simulink model "Limpert_Ex71"  (R2022a)
settings: Solver=FixedStepAuto  StartTime=0.0  StopTime=5  FixedStep=0.001  RelTol=1e-3
settings Model: Creator=roger  LastModifiedBy=wenis

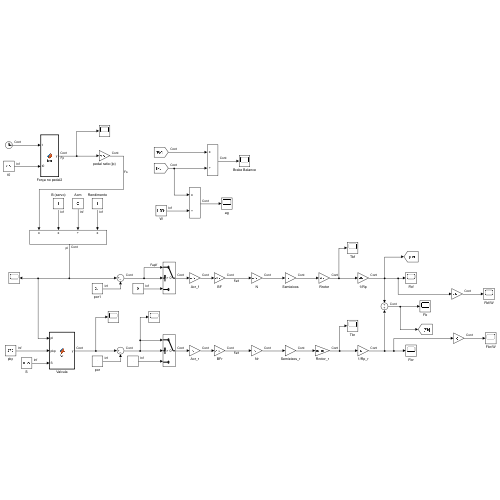
[thumbnail: Simulink's stored preview of the top-level diagram]
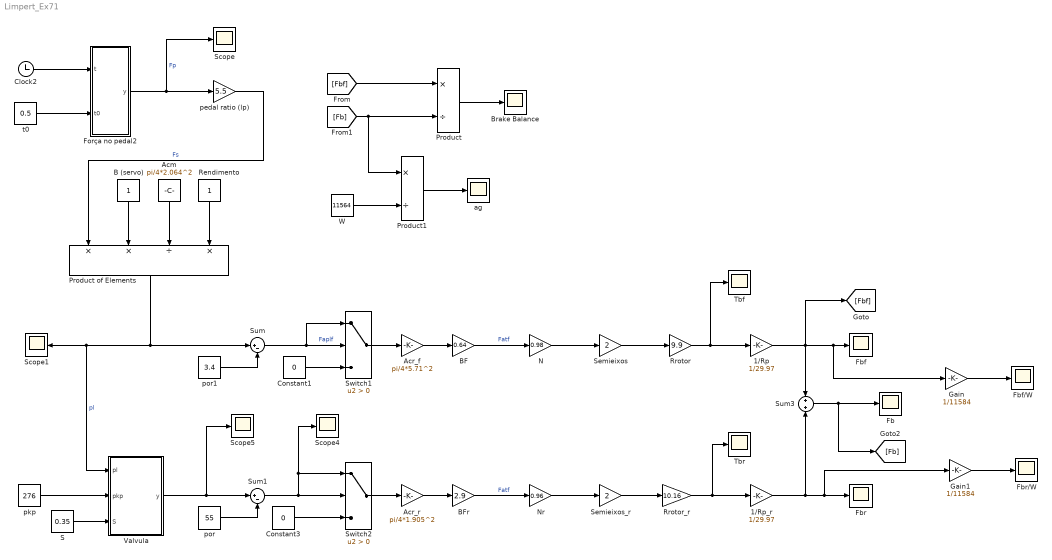
== system Limpert_Ex71 ==
  1/Rp : Gain  Gain=1/29.97
  1/Rp_r : Gain  Gain=1/29.97
  Acm : Constant  Value=pi/4*2.064^2
  Acr_f : Gain  Gain=pi/4*5.71^2
  Acr_r : Gain  Gain=pi/4*1.905^2
  B (servo) : Constant
  BF : Gain  Gain=0.64
  BFr : Gain  Gain=2.9
  Brake Balance : Scope
  Clock2 : Clock
  Constant1 : Constant  Value=0
  Constant3 : Constant  Value=0
  Fb : Scope
  Fbf : Scope
  Fbf/W : Scope
  Fbr : Scope
  Fbr/W : Scope
  Força no pedal2 : MATLAB Function  TreatAsAtomicUnit=on
  Gain : Gain  Gain=1/11584
  Gain1 : Gain  Gain=1/11584
  N : Gain  Gain=0.98
  Nr : Gain  Gain=0.96
  Product : Product  Inputs=*/
  Product of Elements : Product  Inputs=**/*
  Product1 : Product  Inputs=*/
  Rendimento : Constant
  Rrotor : Gain  Gain=9.9
  Rrotor_r : Gain  Gain=10.16
  S : Constant  Value=0.35
  Scope{,1,4..5} (4 alike) : Scope
  Semieixos : Gain  Gain=2
  Semieixos_r : Gain  Gain=2
  Sum : Sum  Inputs=|+-
  Sum1 : Sum  Inputs=|+-
  Sum3 : Sum
  Switch1 : Switch  Criteria=u2 > Threshold  SaturateOnIntegerOverflow=off  InputSameDT=off
  Switch2 : Switch  Criteria=u2 > Threshold  SaturateOnIntegerOverflow=off  InputSameDT=off
  Tbf : Scope
  Tbr : Scope
  Valvula : MATLAB Function  TreatAsAtomicUnit=on
  W : Constant  Value=11564
  ag : Scope
  pedal ratio (lp) : Gain  Gain=5.5
  pkp : Constant  Value=276
  por : Constant  Value=55
  por1 : Constant  Value=3.4
  t0 : Constant  Value=0.5
  wires:
  pedal ratio (lp)/1 -> Product of Elements/1  "Fs"
  B (servo)/1 -> Product of Elements/2
  Acm/1 -> Product of Elements/3
  Rendimento/1 -> Product of Elements/4
  pkp/1 -> Valvula/2(pkp)
  Sum/1 -> Switch1/1, Switch1/2  "Faplf"
  Acr_f/1 -> BF/1
  BF/1 -> N/1  "Fatf"
  N/1 -> Semieixos/1
  Semieixos/1 -> Rrotor/1
  Rrotor/1 -> Tbf/1, 1/Rp/1
  1/Rp/1 -> [Fbf], Sum3/1, Gain/1, Fbf/1
  1/Rp_r/1 -> Sum3/2, Gain1/1, Fbr/1
  Rrotor_r/1 -> 1/Rp_r/1, Tbr/1
  Semieixos_r/1 -> Rrotor_r/1
  Nr/1 -> Semieixos_r/1
  BFr/1 -> Nr/1  "Fatf"
  Acr_r/1 -> BFr/1
  Sum1/1 -> Switch2/2, Switch2/1, Scope4/1
  Sum3/1 -> [Fb], Fb/1
  S/1 -> Valvula/3(S)
  Valvula/1(y) -> Sum1/1, Scope5/1
  Constant3/1 -> Switch2/3
  por/1 -> Sum1/2
  Switch2/1 -> Acr_r/1
  por1/1 -> Sum/2
  Switch1/1 -> Acr_f/1
  Constant1/1 -> Switch1/3
  Product of Elements/1 -> Scope1/1, Valvula/1(pl), Sum/1  "pl"
  Clock2/1 -> Força no pedal2/1(t)
  t0/1 -> Força no pedal2/2(t0)
  Força no pedal2/1(y) -> Scope/1, pedal ratio (lp)/1  "Fp"
  [Fbf] -> Product/1
  [Fb] -> Product1/1, Product/2
  Product/1 -> Brake Balance/1
  W/1 -> Product1/2
  Product1/1 -> ag/1
  Gain/1 -> Fbf/W/1
  Gain1/1 -> Fbr/W/1

== matlab function Limpert_Ex71/Valvula ==
  data: pl input; y output; pkp input; S input
function y = fcn(pl, pkp, S)



if pl <= pkp
    y = pl;
else
    y = pkp + S*(pl-pkp);
end

end

== matlab function Limpert_Ex71/Força no pedal2 ==
  data: t input; y output; t0 input
function y = fcn(t, t0)


if t<=t0
    y=0;
else
    y = 200*(t-t0);
end
